simulink model "GTA_PCMFirmware"  (Simulink 7.8)
settings: Solver=FixedStepDiscrete  StartTime=0.0  StopTime=10.0  RelTol=1e-3
PreLoadFcn:
  | try, eval([bdroot '_setup']); catch, eval('model_setup', ''); end
InitFcn:
  | try, eval([bdroot '_setup']); catch, eval('model_setup', ''); end
undefined symbols (not defined in the file): fndFwd, fndNeut, fndRev, FWDlockout, GCM, keySwIgn2, motohawk_build_version, motohawk_trunc_name, motohawk_vardec_path, REVlockout
libraries: MotoHawk_lib x313, simulink x47, GTA_Library x13
(part 5 of 7)

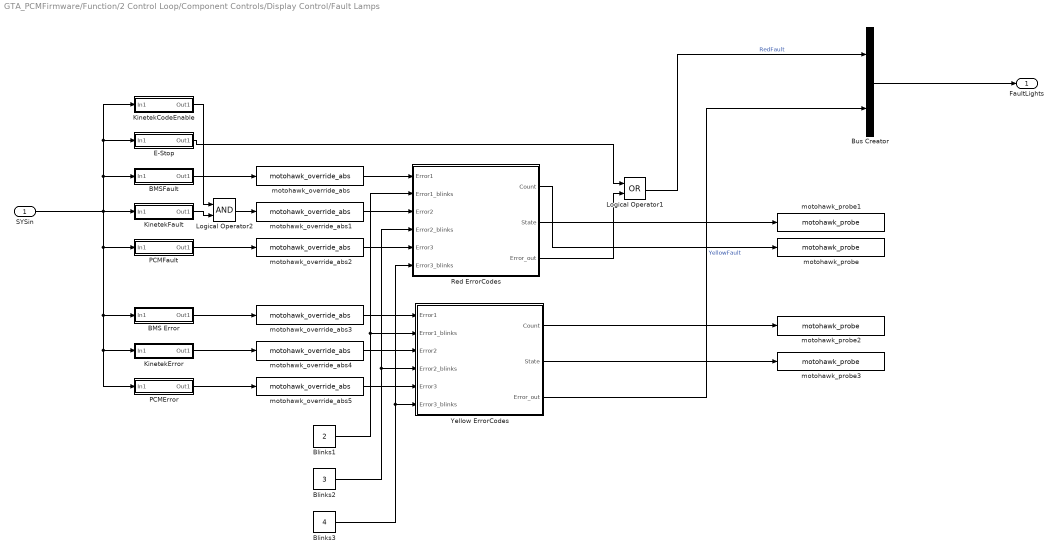
== system GTA_PCMFirmware/Function/2 Control Loop/Component Controls/Display Control/Fault Lamps ==
  SYSin : Inport
  BMS Error : Subsystem
  BMSFault : Subsystem
  Blinks1 : Constant  Value=2
  Blinks2 : Constant  Value=3
  Blinks3 : Constant  Value=4
  Bus Creator : BusCreator  Inputs=2
  E-Stop : Subsystem
  KinetekCodeEnable : Subsystem
  KinetekError : Subsystem
  KinetekFault : Subsystem
  Logical Operator1 : Logic  Operator=OR  AllPortsSameDT=off  OutDataTypeStr=boolean
  Logical Operator2 : Logic  AllPortsSameDT=off  OutDataTypeStr=boolean
  PCMError : Subsystem
  PCMFault : Subsystem
  Red ErrorCodes : Stateflow chart  TreatAsAtomicUnit=on
  Yellow ErrorCodes : Stateflow chart  TreatAsAtomicUnit=on
  motohawk_override_abs : MotoHawk_lib/Calibration & Probing Blocks/motohawk_override_abs  parent_name='BMSfltDBG'  parent_val=0  show_more=off  name_source=Use Parameter  parent_read_level=1  parent_override_level=1  view_as=Number  enum_struct={'Disabled', 'Enabled'}  use_help_units=off  parent_help=''  parent_units=''  use_min_max=off  parent_min=-inf  parent_max=inf  use_precision=off  parent_precision=''  parent_gain=1  parent_offset=0  parent_exp=1  use_mototune_group=off  parent_group=motohawk_vardec_path(gcb)
  motohawk_override_abs1 : MotoHawk_lib/Calibration & Probing Blocks/motohawk_override_abs  parent_name='KINETEKfltDBG'  parent_val=0  show_more=off  name_source=Use Parameter  parent_read_level=1  parent_override_level=1  view_as=Number  enum_struct={'Disabled', 'Enabled'}  use_help_units=off  parent_help=''  parent_units=''  use_min_max=off  parent_min=-inf  parent_max=inf  use_precision=off  parent_precision=''  parent_gain=1  parent_offset=0  parent_exp=1  use_mototune_group=off  parent_group=motohawk_vardec_path(gcb)
  motohawk_override_abs2 : MotoHawk_lib/Calibration & Probing Blocks/motohawk_override_abs  parent_name='PCMfltDBG'  parent_val=0  show_more=off  name_source=Use Parameter  parent_read_level=1  parent_override_level=1  view_as=Number  enum_struct={'Disabled', 'Enabled'}  use_help_units=off  parent_help=''  parent_units=''  use_min_max=off  parent_min=-inf  parent_max=inf  use_precision=off  parent_precision=''  parent_gain=1  parent_offset=0  parent_exp=1  use_mototune_group=off  parent_group=motohawk_vardec_path(gcb)
  motohawk_override_abs3 : MotoHawk_lib/Calibration & Probing Blocks/motohawk_override_abs  parent_name='BMSerrDBG'  parent_val=0  show_more=off  name_source=Use Parameter  parent_read_level=1  parent_override_level=1  view_as=Number  enum_struct={'Disabled', 'Enabled'}  use_help_units=off  parent_help=''  parent_units=''  use_min_max=off  parent_min=-inf  parent_max=inf  use_precision=off  parent_precision=''  parent_gain=1  parent_offset=0  parent_exp=1  use_mototune_group=off  parent_group=motohawk_vardec_path(gcb)
  motohawk_override_abs4 : MotoHawk_lib/Calibration & Probing Blocks/motohawk_override_abs  parent_name='KINETEKerrDBG'  parent_val=0  show_more=off  name_source=Use Parameter  parent_read_level=1  parent_override_level=1  view_as=Number  enum_struct={'Disabled', 'Enabled'}  use_help_units=off  parent_help=''  parent_units=''  use_min_max=off  parent_min=-inf  parent_max=inf  use_precision=off  parent_precision=''  parent_gain=1  parent_offset=0  parent_exp=1  use_mototune_group=off  parent_group=motohawk_vardec_path(gcb)
  motohawk_override_abs5 : MotoHawk_lib/Calibration & Probing Blocks/motohawk_override_abs  parent_name='PCMerrDBG'  parent_val=0  show_more=off  name_source=Use Parameter  parent_read_level=1  parent_override_level=1  view_as=Number  enum_struct={'Disabled', 'Enabled'}  use_help_units=off  parent_help=''  parent_units=''  use_min_max=off  parent_min=-inf  parent_max=inf  use_precision=off  parent_precision=''  parent_gain=1  parent_offset=0  parent_exp=1  use_mototune_group=off  parent_group=motohawk_vardec_path(gcb)
  motohawk_probe : MotoHawk_lib/Calibration & Probing Blocks/motohawk_probe  nam='Red_count'  show_more=off  name_source=Use Parameter  read_level=1  view_as=Number  enum_struct={'Disabled', 'Enabled'}  vector_style=Wide Row  use_help_units=off  help=''  units=''  use_header_enum=off  row_header_enum={}  col_header_enum={}  use_min_max=off  min_val=-inf  max_val=inf  use_precision=off  precision=''  gain=1  offset=0  exp=1  use_mototune_group=off  mototune_group=motohawk_vardec_path(gcb)
  motohawk_probe1 : MotoHawk_lib/Calibration & Probing Blocks/motohawk_probe  nam='Red_state'  show_more=off  name_source=Use Parameter  read_level=1  view_as=Number  enum_struct={'Disabled', 'Enabled'}  vector_style=Wide Row  use_help_units=off  help=''  units=''  use_header_enum=off  row_header_enum={}  col_header_enum={}  use_min_max=off  min_val=-inf  max_val=inf  use_precision=off  precision=''  gain=1  offset=0  exp=1  use_mototune_group=off  mototune_group=motohawk_vardec_path(gcb)
  motohawk_probe2 : MotoHawk_lib/Calibration & Probing Blocks/motohawk_probe  nam='Yellow_count'  show_more=off  name_source=Use Parameter  read_level=1  view_as=Number  enum_struct={'Disabled', 'Enabled'}  vector_style=Wide Row  use_help_units=off  help=''  units=''  use_header_enum=off  row_header_enum={}  col_header_enum={}  use_min_max=off  min_val=-inf  max_val=inf  use_precision=off  precision=''  gain=1  offset=0  exp=1  use_mototune_group=off  mototune_group=motohawk_vardec_path(gcb)
  motohawk_probe3 : MotoHawk_lib/Calibration & Probing Blocks/motohawk_probe  nam='Yellow_state'  show_more=off  name_source=Use Parameter  read_level=1  view_as=Number  enum_struct={'Disabled', 'Enabled'}  vector_style=Wide Row  use_help_units=off  help=''  units=''  use_header_enum=off  row_header_enum={}  col_header_enum={}  use_min_max=off  min_val=-inf  max_val=inf  use_precision=off  precision=''  gain=1  offset=0  exp=1  use_mototune_group=off  mototune_group=motohawk_vardec_path(gcb)
  FaultLights : Outport
  wires:
  SYSin/1 -> KinetekFault/1(In1), BMSFault/1(In1), E-Stop/1(In1), KinetekCodeEnable/1(In1), PCMFault/1(In1), BMS Error/1(In1), KinetekError/1(In1), PCMError/1(In1)
  Blinks1/1 -> Red ErrorCodes/2(Error1_blinks), Yellow ErrorCodes/2(Error1_blinks)
  Blinks2/1 -> Red ErrorCodes/4(Error2_blinks), Yellow ErrorCodes/4(Error2_blinks)
  Blinks3/1 -> Red ErrorCodes/6(Error3_blinks), Yellow ErrorCodes/6(Error3_blinks)
  BMSFault/1(Out1) -> motohawk_override_abs/1
  PCMFault/1(Out1) -> motohawk_override_abs2/1
  BMS Error/1(Out1) -> motohawk_override_abs3/1
  KinetekError/1(Out1) -> motohawk_override_abs4/1
  PCMError/1(Out1) -> motohawk_override_abs5/1
  E-Stop/1(Out1) -> Logical Operator1/1
  Yellow ErrorCodes/3(Error_out) -> Bus Creator/2  "YellowFault"
  Logical Operator1/1 -> Bus Creator/1  "RedFault"
  Red ErrorCodes/3(Error_out) -> Logical Operator1/2
  KinetekFault/1(Out1) -> Logical Operator2/2
  KinetekCodeEnable/1(Out1) -> Logical Operator2/1
  Logical Operator2/1 -> motohawk_override_abs1/1
  Yellow ErrorCodes/2(State) -> motohawk_probe3/1
  Yellow ErrorCodes/1(Count) -> motohawk_probe2/1
  Red ErrorCodes/2(State) -> motohawk_probe1/1
  Red ErrorCodes/1(Count) -> motohawk_probe/1
  motohawk_override_abs/1 -> Red ErrorCodes/1(Error1)
  motohawk_override_abs1/1 -> Red ErrorCodes/3(Error2)
  motohawk_override_abs2/1 -> Red ErrorCodes/5(Error3)
  motohawk_override_abs3/1 -> Yellow ErrorCodes/1(Error1)
  motohawk_override_abs4/1 -> Yellow ErrorCodes/3(Error2)
  motohawk_override_abs5/1 -> Yellow ErrorCodes/5(Error3)
  Bus Creator/1 -> FaultLights/1

== system GTA_PCMFirmware/Function/2 Control Loop/Component Controls/Display Control/Gearbox Display ==
  SYSin : Inport
  MotorControl : Inport  Port=2
  Bus Selector : BusSelector  OutputSignals=fndOutput
  Bus Selector1 : BusSelector  OutputSignals=ModeControl.StatusBits.DriveMode
  Data Type Conversion : DataTypeConversion  OutDataTypeStr=boolean
  Drive : Constant  Value=hex2dec('B')  OutDataTypeStr=uint16
  DriveOrRev : Constant  OutDataTypeStr=boolean
  Flash Neutral : Constant  Value=hex2dec('C')  OutDataTypeStr=uint16
  Logical Operator : Logic  Operator=NOT  AllPortsSameDT=off  OutDataTypeStr=boolean
  Logical Operator1 : Logic  Inputs=3  AllPortsSameDT=off  OutDataTypeStr=boolean
  Multiport Switch : MultiPortSwitch  DataPortOrder=Zero-based contiguous  Inputs=4  zeroidx=on
  Multiport Switch1 : MultiPortSwitch  DataPortOrder=Zero-based contiguous  Inputs=4  zeroidx=on
  Multiport Switch2 : MultiPortSwitch  DataPortOrder=Zero-based contiguous  Inputs=2  zeroidx=on
  Neutral : Constant  Value=hex2dec('C')  OutDataTypeStr=uint16
  Neutral1 : Constant  Value=0  OutDataTypeStr=boolean
  NotValid : Constant  Value=hex2dec('F')  OutDataTypeStr=uint16
  Pulse Generator : DiscretePulseGenerator  Period=250  PulseWidth=125  SampleTime=-1
  Reverse : Constant  Value=hex2dec('D')  OutDataTypeStr=uint16
  GboxPos : Outport
  wires:
  MotorControl/1 -> Bus Selector/1
  Bus Selector/1 -> Multiport Switch/1, Multiport Switch1/1  "<fndOutput>"
  Neutral/1 -> Multiport Switch/2
  NotValid/1 -> Multiport Switch/5
  Multiport Switch/1 -> Multiport Switch2/2  "GearboxPositionIPC"
  Reverse/1 -> Multiport Switch/3
  Drive/1 -> Multiport Switch/4
  DriveOrRev/1 -> Multiport Switch1/3, Multiport Switch1/4
  Neutral1/1 -> Multiport Switch1/2, Multiport Switch1/5
  Bus Selector1/1 -> Logical Operator/1  "<DriveMode>"
  Multiport Switch1/1 -> Logical Operator1/1
  Logical Operator/1 -> Logical Operator1/2
  Pulse Generator/1 -> Data Type Conversion/1
  Logical Operator1/1 -> Multiport Switch2/1
  Flash Neutral/1 -> Multiport Switch2/3
  Multiport Switch2/1 -> GboxPos/1  "GearboxPositionIPC"
  Data Type Conversion/1 -> Logical Operator1/3
  SYSin/1 -> Bus Selector1/1

== system GTA_PCMFirmware/Function/2 Control Loop/Component Controls/Display Control/ReadyLight ==
  SYSin : Inport
  Bus Selector1 : BusSelector  OutputSignals=ReadyState,ModeControl.StatusBits.ReadyOk
  Logical Operator : Logic  AllPortsSameDT=off  OutDataTypeStr=boolean
  ReadyLight : Outport
  wires:
  SYSin/1 -> Bus Selector1/1
  Bus Selector1/1 -> Logical Operator/1  "<ReadyState>"
  Bus Selector1/2 -> Logical Operator/2  "<ReadyOk>"
  Logical Operator/1 -> ReadyLight/1

== system GTA_PCMFirmware/Function/2 Control Loop/Component Controls/Display Control/Vehicle Speed ==
  SYSin : Inport
  Bus Selector1 : BusSelector  OutputSignals=BUS.Input Bus.CANin.Motor Controller.KinVoltSpeed.SpeedLPF
  RPMtoInperMin : Gain  Gain=33/4925  OutDataTypeStr=single
  Out1 : Outport
  wires:
  SYSin/1 -> Bus Selector1/1
  Bus Selector1/1 -> RPMtoInperMin/1  "<SpeedLPF>"
  RPMtoInperMin/1 -> Out1/1  "vehSpeed"

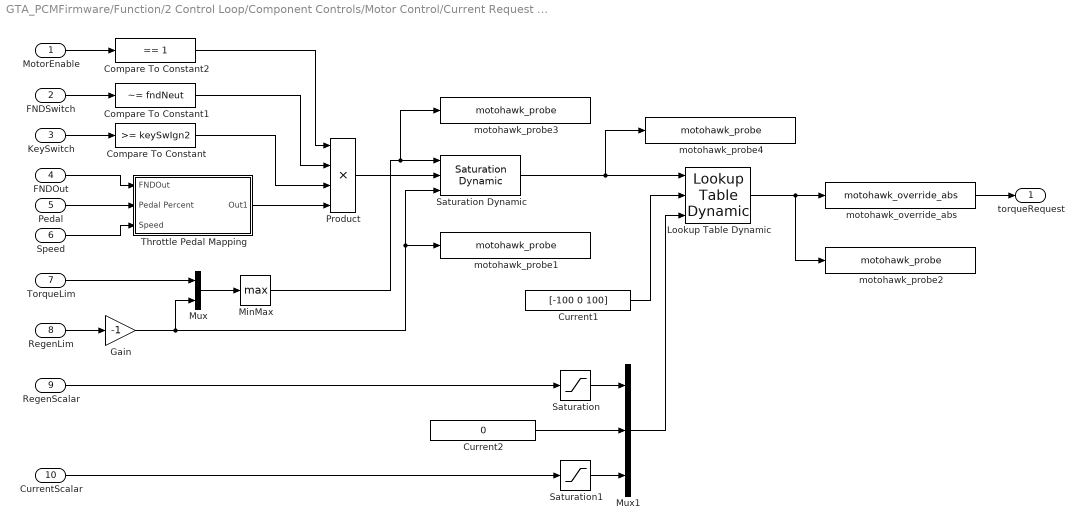
== system GTA_PCMFirmware/Function/2 Control Loop/Component Controls/Motor Control/Current Request Algorithm ==
  MotorEnable : Inport
  "FNDSwitch " : Inport  Port=2
  KeySwitch : Inport  Port=3
  FNDOut : Inport  Port=4
  "Pedal " : Inport  Port=5
  Speed : Inport  Port=6
  "TorqueLim " : Inport  Port=7
  RegenLim : Inport  Port=8
  RegenScalar : Inport  Port=9  OutDataTypeStr=single
  CurrentScalar : Inport  Port=10  OutDataTypeStr=single
  Compare To Constant : simulink/Logic and Bit Operations/Compare To Constant  relop=>=  const=keySwIgn2  OutDataTypeStr=uint8
  Compare To Constant1 : simulink/Logic and Bit Operations/Compare To Constant  relop=~=  const=fndNeut  OutDataTypeStr=uint8
  Compare To Constant2 : simulink/Logic and Bit Operations/Compare To Constant  relop===  const=1  OutDataTypeStr=uint8
  Current1 : Constant  Value=[-100 0 100]  OutDataTypeStr=single
  Current2 : Constant  Value=0  OutDataTypeStr=single
  Gain : Gain  Gain=-1
  Lookup Table Dynamic : simulink/Lookup Tables/Lookup Table Dynamic  LookUpMeth=Interpolation-Use End Values  OutDataTypeStr=fixdt('single')  OutputDataTypeScalingMode=Specify via dialog  OutDataType=fixdt('single')  OutScaling=[]  DoSatur=off
  MinMax : MinMax  Function=max
  Mux : Mux  Inputs=2
  Mux1 : Mux  Inputs=3
  Product : Product  Inputs=4  OutDataTypeStr=single  RndMeth=Zero
  Saturation : Saturate  UpperLimit=0  LowerLimit=-1000  OutDataTypeStr=single
  Saturation Dynamic : simulink/Discontinuities/Saturation Dynamic  OutMin=[]  OutMax=[]  OutDataTypeStr=Inherit: Same as second input  OutDataType=fixdt(1, 16)  OutScaling=2^-10  DoSatur=off
  Saturation1 : Saturate  UpperLimit=1000  LowerLimit=0  OutDataTypeStr=single
  Throttle Pedal Mapping : Subsystem
  motohawk_override_abs : MotoHawk_lib/Calibration & Probing Blocks/motohawk_override_abs  parent_name='Motor_Current_Override'  parent_val=0  show_more=on  name_source=Use Parameter  parent_read_level=1  parent_override_level=1  view_as=Number  enum_struct={'Disabled', 'Enabled'}  use_help_units=off  parent_help=''  parent_units=''  use_min_max=off  parent_min=-inf  parent_max=inf  use_precision=off  parent_precision=''  parent_gain=1  parent_offset=0  parent_exp=1  use_mototune_group=off  parent_group=motohawk_vardec_path(gcb)
  motohawk_probe1 : MotoHawk_lib/Calibration & Probing Blocks/motohawk_probe  nam='LowSatLimit'  show_more=on  name_source=Use Parameter  read_level=1  view_as=Number  enum_struct={'Disabled', 'Enabled'}  vector_style=Wide Row  use_help_units=off  help=''  units=''  use_header_enum=off  row_header_enum={}  col_header_enum={}  use_min_max=off  min_val=-inf  max_val=inf  use_precision=off  precision=''  gain=1  offset=0  exp=1  use_mototune_group=off  mototune_group=motohawk_vardec_path(gcb)
  motohawk_probe2 : MotoHawk_lib/Calibration & Probing Blocks/motohawk_probe  nam='Motor_Current_Output'  show_more=on  name_source=Use Parameter  read_level=1  view_as=Number  enum_struct={'Disabled', 'Enabled'}  vector_style=Wide Row  use_help_units=off  help=''  units=''  use_header_enum=off  row_header_enum={}  col_header_enum={}  use_min_max=off  min_val=-inf  max_val=inf  use_precision=off  precision=''  gain=1  offset=0  exp=1  use_mototune_group=off  mototune_group=motohawk_vardec_path(gcb)
  motohawk_probe3 : MotoHawk_lib/Calibration & Probing Blocks/motohawk_probe  nam='HighSatLimit'  show_more=on  name_source=Use Parameter  read_level=1  view_as=Number  enum_struct={'Disabled', 'Enabled'}  vector_style=Wide Row  use_help_units=off  help=''  units=''  use_header_enum=off  row_header_enum={}  col_header_enum={}  use_min_max=off  min_val=-inf  max_val=inf  use_precision=off  precision=''  gain=1  offset=0  exp=1  use_mototune_group=off  mototune_group=motohawk_vardec_path(gcb)
  motohawk_probe4 : MotoHawk_lib/Calibration & Probing Blocks/motohawk_probe  nam='PedalLookupOutPercent'  show_more=on  name_source=Use Parameter  read_level=1  view_as=Number  enum_struct={'Disabled', 'Enabled'}  vector_style=Wide Row  use_help_units=off  help=''  units=''  use_header_enum=off  row_header_enum={}  col_header_enum={}  use_min_max=off  min_val=-inf  max_val=inf  use_precision=off  precision=''  gain=1  offset=0  exp=1  use_mototune_group=off  mototune_group=motohawk_vardec_path(gcb)
  torqueRequest : Outport
  wires:
  "TorqueLim "/1 -> Mux/1
  KeySwitch/1 -> Compare To Constant/1
  "FNDSwitch "/1 -> Compare To Constant1/1
  motohawk_override_abs/1 -> torqueRequest/1
  FNDOut/1 -> Throttle Pedal Mapping/1(FNDOut)
  "Pedal "/1 -> Throttle Pedal Mapping/2(Pedal Percent)
  Speed/1 -> Throttle Pedal Mapping/3(Speed)
  Throttle Pedal Mapping/1(Out1) -> Product/4
  Compare To Constant/1 -> Product/3
  Compare To Constant1/1 -> Product/2
  Product/1 -> Saturation Dynamic/2
  Mux/1 -> MinMax/1
  MinMax/1 -> motohawk_probe3/1, Saturation Dynamic/1
  Lookup Table Dynamic/1 -> motohawk_override_abs/1, motohawk_probe2/1
  Saturation Dynamic/1 -> Lookup Table Dynamic/1, motohawk_probe4/1
  RegenLim/1 -> Gain/1
  Current1/1 -> Lookup Table Dynamic/2
  Saturation/1 -> Mux1/1
  Current2/1 -> Mux1/2
  Saturation1/1 -> Mux1/3
  Mux1/1 -> Lookup Table Dynamic/3
  RegenScalar/1 -> Saturation/1
  Gain/1 -> Mux/2, Saturation Dynamic/3, motohawk_probe1/1
  MotorEnable/1 -> Compare To Constant2/1
  Compare To Constant2/1 -> Product/1
  CurrentScalar/1 -> Saturation1/1

== system GTA_PCMFirmware/Function/2 Control Loop/Component Controls/Motor Control/Direction Lockout ==
  " FNDSw" : Inport
  " Speed" : Inport  Port=2
  Forward : simulink/Logic and Bit Operations/Compare To Constant  relop===  const=fndRev  OutDataTypeStr=boolean
  Fwd Lockout : simulink/Logic and Bit Operations/Compare To Constant  relop=>=  const=FWDlockout  OutDataTypeStr=boolean
  Fwd while Rev : Logic  AllPortsSameDT=off  OutDataTypeStr=boolean
  Gain : Gain  OutDataTypeStr=uint16
  Multiport Switch : MultiPortSwitch  DataPortOrder=Specify indices  Inputs=2  DataPortIndices={0,1}  zeroidx=off
  Neutral : Constant  Value=fndNeut
  Neutral command : Logic  Operator=OR  AllPortsSameDT=off  OutDataTypeStr=boolean
  Rev Lockout : simulink/Logic and Bit Operations/Compare To Constant  relop=<=  const=REVlockout  OutDataTypeStr=boolean
  Rev while Fwd : Logic  AllPortsSameDT=off  OutDataTypeStr=boolean
  Reverse : simulink/Logic and Bit Operations/Compare To Constant  relop===  const=fndFwd  OutDataTypeStr=boolean
  " FNDOut" : Outport
  wires:
  " FNDSw"/1 -> Gain/1
  Gain/1 -> Forward/1, Reverse/1, Multiport Switch/2  "fndOutput"
  " Speed"/1 -> Fwd Lockout/1, Rev Lockout/1
  Forward/1 -> Rev while Fwd/1
  Fwd Lockout/1 -> Rev while Fwd/2
  Reverse/1 -> Fwd while Rev/1
  Rev Lockout/1 -> Fwd while Rev/2
  Fwd while Rev/1 -> Neutral command/2
  Rev while Fwd/1 -> Neutral command/1
  Multiport Switch/1 -> " FNDOut"/1  "fndOutput"
  Neutral/1 -> Multiport Switch/3
  Neutral command/1 -> Multiport Switch/1

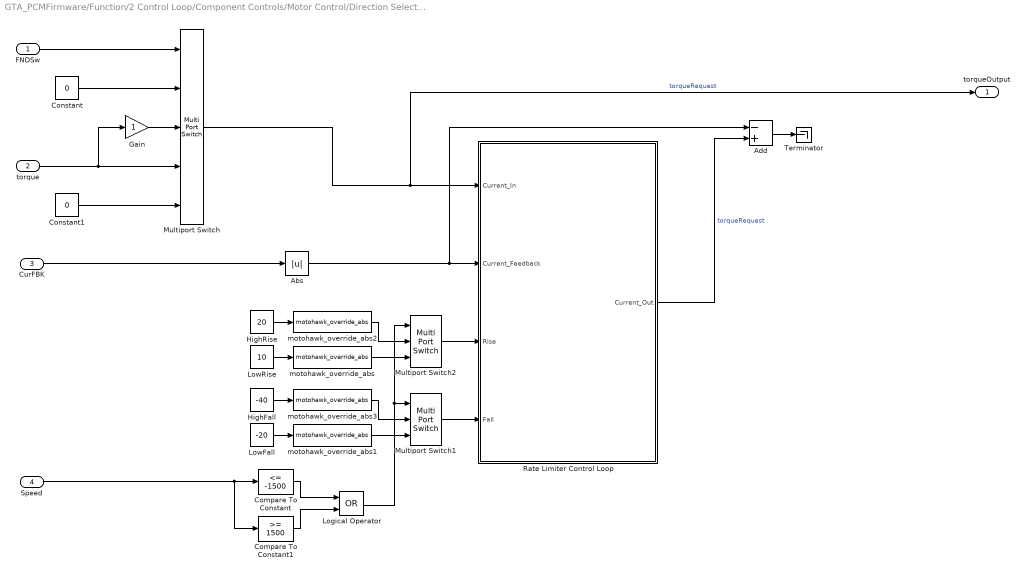
== system GTA_PCMFirmware/Function/2 Control Loop/Component Controls/Motor Control/Direction Selector & Control Loop ==
  " FNDSw" : Inport
  " torque" : Inport  Port=2
  CurFBK : Inport  Port=3
  Speed : Inport  Port=4
  Abs : Abs
  Add : Sum  Inputs=-+
  Compare To Constant : simulink/Logic and Bit Operations/Compare To Constant  relop=<=  const=-1500  OutDataTypeStr=boolean
  Compare To Constant1 : simulink/Logic and Bit Operations/Compare To Constant  relop=>=  const=1500  OutDataTypeStr=boolean
  Constant : Constant  Value=0
  Constant1 : Constant  Value=0
  Gain : Gain
  HighFall : Constant  Value=-40
  HighRise : Constant  Value=20
  Logical Operator : Logic  Operator=OR  AllPortsSameDT=off  OutDataTypeStr=boolean
  LowFall : Constant  Value=-20
  LowRise : Constant  Value=10
  Multiport Switch : MultiPortSwitch  DataPortOrder=Zero-based contiguous  Inputs=4  zeroidx=on
  Multiport Switch1 : MultiPortSwitch  DataPortOrder=Specify indices  DataPortIndices={1,0}  zeroidx=off
  Multiport Switch2 : MultiPortSwitch  DataPortOrder=Specify indices  DataPortIndices={1,0}  zeroidx=off
  Rate Limiter Control Loop : Stateflow chart  TreatAsAtomicUnit=on
  Terminator : Terminator
  motohawk_override_abs : MotoHawk_lib/Calibration & Probing Blocks/motohawk_override_abs  parent_name='RateLimitRiseLow'  parent_val=10  show_more=off  name_source=Use Parameter  parent_read_level=1  parent_override_level=1  view_as=Number  enum_struct={'Disabled', 'Enabled'}  use_help_units=off  parent_help=''  parent_units=''  use_min_max=off  parent_min=-inf  parent_max=inf  use_precision=off  parent_precision=''  parent_gain=1  parent_offset=0  parent_exp=1  use_mototune_group=off  parent_group=motohawk_vardec_path(gcb)
  motohawk_override_abs1 : MotoHawk_lib/Calibration & Probing Blocks/motohawk_override_abs  parent_name='RateLimitFallLow'  parent_val=0  show_more=off  name_source=Use Parameter  parent_read_level=1  parent_override_level=1  view_as=Number  enum_struct={'Disabled', 'Enabled'}  use_help_units=off  parent_help=''  parent_units=''  use_min_max=off  parent_min=-inf  parent_max=inf  use_precision=off  parent_precision=''  parent_gain=1  parent_offset=0  parent_exp=1  use_mototune_group=off  parent_group=motohawk_vardec_path(gcb)
  motohawk_override_abs2 : MotoHawk_lib/Calibration & Probing Blocks/motohawk_override_abs  parent_name='RateLimitRiseHigh'  parent_val=10  show_more=off  name_source=Use Parameter  parent_read_level=1  parent_override_level=1  view_as=Number  enum_struct={'Disabled', 'Enabled'}  use_help_units=off  parent_help=''  parent_units=''  use_min_max=off  parent_min=-inf  parent_max=inf  use_precision=off  parent_precision=''  parent_gain=1  parent_offset=0  parent_exp=1  use_mototune_group=off  parent_group=motohawk_vardec_path(gcb)
  motohawk_override_abs3 : MotoHawk_lib/Calibration & Probing Blocks/motohawk_override_abs  parent_name='RateLimitFallHigh'  parent_val=0  show_more=off  name_source=Use Parameter  parent_read_level=1  parent_override_level=1  view_as=Number  enum_struct={'Disabled', 'Enabled'}  use_help_units=off  parent_help=''  parent_units=''  use_min_max=off  parent_min=-inf  parent_max=inf  use_precision=off  parent_precision=''  parent_gain=1  parent_offset=0  parent_exp=1  use_mototune_group=off  parent_group=motohawk_vardec_path(gcb)
  torqueOutput : Outport
  wires:
  " FNDSw"/1 -> Multiport Switch/1
  " torque"/1 -> Multiport Switch/4, Gain/1
  Gain/1 -> Multiport Switch/3
  Constant/1 -> Multiport Switch/2
  Constant1/1 -> Multiport Switch/5
  Speed/1 -> Compare To Constant/1, Compare To Constant1/1
  Compare To Constant/1 -> Logical Operator/1
  Compare To Constant1/1 -> Logical Operator/2
  Multiport Switch/1 -> Rate Limiter Control Loop/1(Current_In), torqueOutput/1  "torqueRequest"
  LowFall/1 -> motohawk_override_abs1/1
  LowRise/1 -> motohawk_override_abs/1
  HighRise/1 -> motohawk_override_abs2/1
  HighFall/1 -> motohawk_override_abs3/1
  motohawk_override_abs/1 -> Multiport Switch2/3
  motohawk_override_abs1/1 -> Multiport Switch1/3
  motohawk_override_abs3/1 -> Multiport Switch1/2
  motohawk_override_abs2/1 -> Multiport Switch2/2
  Multiport Switch2/1 -> Rate Limiter Control Loop/3(Rise)
  Multiport Switch1/1 -> Rate Limiter Control Loop/4(Fall)
  Logical Operator/1 -> Multiport Switch2/1, Multiport Switch1/1
  CurFBK/1 -> Abs/1
  Rate Limiter Control Loop/1(Current_Out) -> Add/2  "torqueRequest"
  Abs/1 -> Rate Limiter Control Loop/2(Current_Feedback), Add/1
  Add/1 -> Terminator/1

== system GTA_PCMFirmware/Function/2 Control Loop/Component Controls/Motor Control/Enable ==
  "driveEnable " : Inport
  errorField : Inport  Port=2
  Compare To Constant : simulink/Logic and Bit Operations/Compare To Constant  relop===  const=0  OutDataTypeStr=uint8
  Logical Operator : Logic  AllPortsSameDT=off  OutDataTypeStr=boolean
  Terminator : Terminator
  enable : Outport
  wires:
  Logical Operator/1 -> enable/1  "enable"
  "driveEnable "/1 -> Logical Operator/1, Logical Operator/2
  errorField/1 -> Compare To Constant/1
  Compare To Constant/1 -> Terminator/1

== system GTA_PCMFirmware/Function/2 Control Loop/Mode Control & Ready/Mode Control/Status Bits ==
  ModeState : Inport
  Fault_ID : Inport  Port=2
  HVstate : Inport  Port=3
  ACC2Mode : simulink/Logic and Bit Operations/Compare To Constant  relop=~=  const=0  OutDataTypeStr=uint8
  Bus Creator : BusCreator  Inputs=6
  Compare : simulink/Logic and Bit Operations/Compare To Constant  relop===  const=2  OutDataTypeStr=uint8
  Compare1 : simulink/Logic and Bit Operations/Compare To Constant  relop===  const=1  OutDataTypeStr=uint8
  Compare2 : simulink/Logic and Bit Operations/Compare To Constant  relop===  const=5  OutDataTypeStr=uint8
  Compare3 : simulink/Logic and Bit Operations/Compare To Constant  relop=~=  const=0  OutDataTypeStr=uint8
  Compare4 : simulink/Logic and Bit Operations/Compare To Constant  relop===  const=4  OutDataTypeStr=uint8
  Compare5 : simulink/Logic and Bit Operations/Compare To Constant  relop===  const=2  OutDataTypeStr=uint8
  Logical Operator : Logic  Operator=OR  AllPortsSameDT=off  OutDataTypeStr=boolean
  Terminator : Terminator
  StatusOut : Outport
  wires:
  Bus Creator/1 -> StatusOut/1
  Compare1/1 -> Logical Operator/1
  Compare/1 -> Logical Operator/2
  Logical Operator/1 -> Bus Creator/1  "ChargeMode"
  Compare2/1 -> Bus Creator/2  "DriveMode"
  Fault_ID/1 -> Compare3/1, Compare4/1, Compare5/1
  Compare3/1 -> Bus Creator/3  "FaultMode"
  ModeState/1 -> Compare1/1, Compare/1, Compare2/1, ACC2Mode/1
  Compare4/1 -> Bus Creator/4  "ContactorFault"
  Compare5/1 -> Bus Creator/5  "BatteryFault"
  ACC2Mode/1 -> Bus Creator/6  "ReadyOk"
  HVstate/1 -> Terminator/1

== system GTA_PCMFirmware/Function/2 Control Loop/Safety/Current Limit/RegenLimit ==
  InputBus : Inport
  Bus Creator : BusCreator  Inputs=3
  Cell Temp too high : simulink/Logic and Bit Operations/Compare To Zero  relop===  OutDataTypeStr=uint8
  Cell Temp too low : simulink/Logic and Bit Operations/Compare To Zero  relop===  OutDataTypeStr=uint8
  Cell Voltage limiter : Subsystem
  Current Limiter : Subsystem
  High Cell Temp : Subsystem
  Low Cell Temp : Subsystem
  MinMax : MinMax
  Mux : Mux  Inputs=6
  Pack Voltage Limiter : Subsystem
  SOC Limiter : Subsystem
  Saturation : Saturate  UpperLimit=100  LowerLimit=0  OutDataTypeStr=single
  motohawk_probe : MotoHawk_lib/Calibration & Probing Blocks/motohawk_probe  nam='RegenLimitPerc'  show_more=off  name_source=Use Parameter  read_level=1  view_as=Number  enum_struct={'Disabled', 'Enabled'}  vector_style=Wide Row  use_help_units=off  help=''  units=''  use_header_enum=off  row_header_enum={}  col_header_enum={}  use_min_max=off  min_val=-inf  max_val=inf  use_precision=off  precision=''  gain=1  offset=0  exp=1  use_mototune_group=off  mototune_group=motohawk_vardec_path(gcb)
  Out : Outport
  wires:
  InputBus/1 -> SOC Limiter/1(InputBus), Pack Voltage Limiter/1(InputBus), Current Limiter/1(InputBus), Cell Voltage limiter/1(InputBus), Low Cell Temp/1(InputBus), High Cell Temp/1(InputBus)
  Pack Voltage Limiter/1(PercOut) -> Mux/1
  Current Limiter/1(PercOut) -> Mux/2
  SOC Limiter/1(PercOut) -> Mux/3
  Mux/1 -> Saturation/1
  Bus Creator/1 -> Out/1
  Saturation/1 -> MinMax/1, motohawk_probe/1
  MinMax/1 -> Bus Creator/1  "MaxRegenPerc"
  Cell Temp too low/1 -> Bus Creator/3  "CellRegTempLo"
  Cell Temp too high/1 -> Bus Creator/2  "CellRegTempHi"
  Cell Voltage limiter/1(PercOut) -> Mux/4
  High Cell Temp/1(PercOut) -> Mux/5, Cell Temp too high/1
  Low Cell Temp/1(PercOut) -> Mux/6, Cell Temp too low/1

== system GTA_PCMFirmware/Function/2 Control Loop/Safety/Current Limit/TorqueLimit ==
  InputBus : Inport
  Bus Creator : BusCreator  Inputs=3
  Cell Temp too high : simulink/Logic and Bit Operations/Compare To Zero  relop===  OutDataTypeStr=uint8
  Cell Temp too low : simulink/Logic and Bit Operations/Compare To Zero  relop===  OutDataTypeStr=uint8
  Cell Voltage limiter : Subsystem
  Current Limiter : Subsystem
  High Cell Temp : Subsystem
  Low Cell Temp : Subsystem
  MinMax : MinMax
  Mux : Mux  Inputs=7
  Pack Voltage Limiter : Subsystem
  SOC Limiter : Subsystem
  Saturation : Saturate  UpperLimit=100  LowerLimit=-100  OutDataTypeStr=single
  Speed Limiter : Subsystem
  motohawk_probe : MotoHawk_lib/Calibration & Probing Blocks/motohawk_probe  nam='torqueLimitPerc'  show_more=off  name_source=Use Parameter  read_level=1  view_as=Number  enum_struct={'Disabled', 'Enabled'}  vector_style=Wide Row  use_help_units=off  help=''  units=''  use_header_enum=off  row_header_enum={}  col_header_enum={}  use_min_max=off  min_val=-inf  max_val=inf  use_precision=off  precision=''  gain=1  offset=0  exp=1  use_mototune_group=off  mototune_group=motohawk_vardec_path(gcb)
  Out : Outport
  wires:
  InputBus/1 -> Speed Limiter/1(InputBus), SOC Limiter/1(InputBus), Pack Voltage Limiter/1(InputBus), Current Limiter/1(InputBus), Low Cell Temp/1(InputBus), High Cell Temp/1(InputBus), Cell Voltage limiter/1(InputBus)
  Pack Voltage Limiter/1(PercOut) -> Mux/1
  Current Limiter/1(PercOut) -> Mux/2
  SOC Limiter/1(PercOut) -> Mux/3
  Speed Limiter/1(PercentOut) -> Mux/4
  Cell Voltage limiter/1(PercOut) -> Mux/5
  High Cell Temp/1(PercOut) -> Mux/6, Cell Temp too high/1
  Low Cell Temp/1(PercOut) -> Mux/7, Cell Temp too low/1
  Mux/1 -> Saturation/1
  Bus Creator/1 -> Out/1
  Saturation/1 -> MinMax/1, motohawk_probe/1
  MinMax/1 -> Bus Creator/1  "MaxCurrPerc"
  Cell Temp too low/1 -> Bus Creator/3  "CellDisTempLo"
  Cell Temp too high/1 -> Bus Creator/2  "CellDisTempHi"

== system GTA_PCMFirmware/Function/2 Control Loop/Safety/Faults/BatteryFault ==
  InputBus : Inport
  {1,4..5,7} (4 alike) : RelationalOperator  OutDataTypeStr=boolean
  {2..3,6,8} (4 alike) : RelationalOperator  Operator=<=  OutDataTypeStr=boolean
  Bus Creator : BusCreator  Inputs=2
  Bus Creator1 : BusCreator  Inputs=8
  Bus Selector : BusSelector  OutputSignals=Input Bus.CANin.BMS.csCellInfo.PackVoltage,Input Bus.Limits.BattLimits.MaxPackVoltage,Input Bus.CANin.BMS.csCellInfo.PackVoltage,Input Bus.Limits.BattLimits.MinPackVoltage,Input Bus.CANin.BMS.csInfo.csCurrent,Input Bus.Limits.BattLimits.CurrentLimit,Input Bus.CANin.BMS.csInfo.csCurrent,Input Bus.Limits.BattLimits.RegenLimit,Input Bus.CANin.BMS.csCellInfo.HighCellValue,Input Bus.Limits.BattLimits.MaxCellVoltage,Input Bus.CANin.BMS.csCellInfo.LowCellValue,Input Bus.Limits.BattLimits.MinCellVoltage,Input Bus.CANin.BMS.csCellTemps.HighCellTemp,Input Bus.Limits.BattLimits.BFmaxCellTemp,Input Bus.CANin.BMS.csCellTemps.LowCellTemp,Input Bus.Limits.BattLimits.BFminCellTemp
  Filter : Subsystem
  Logical Operator : Logic  Operator=OR  Inputs=1  AllPortsSameDT=off  OutDataTypeStr=boolean
  Mux : Mux  Inputs=8
  motohawk_probe : MotoHawk_lib/Calibration & Probing Blocks/motohawk_probe  nam='battFault'  show_more=off  name_source=Use Parameter  read_level=1  view_as=Number  enum_struct={'Disabled', 'Enabled'}  vector_style=Wide Row  use_help_units=off  help=''  units=''  use_header_enum=off  row_header_enum={}  col_header_enum={}  use_min_max=off  min_val=-inf  max_val=inf  use_precision=off  precision=''  gain=1  offset=0  exp=1  use_mototune_group=off  mototune_group=motohawk_vardec_path(gcb)
  BatteryFault : Outport
  wires:
  InputBus/1 -> Bus Selector/1
  Bus Selector/6 -> 3/2  "<CurrentLimit>"
  Bus Selector/8 -> 4/2  "<RegenLimit>"
  Bus Selector/9 -> 5/1  "<HighCellValue>"
  Bus Selector/10 -> 5/2  "<MaxCellVoltage>"
  Bus Selector/11 -> 6/1  "<LowCellValue>"
  Bus Selector/12 -> 6/2  "<MinCellVoltage>"
  Bus Selector/2 -> 1/2  "<MaxPackVoltage>"
  Bus Selector/4 -> 2/2  "<MinPackVoltage>"
  1/1 -> Mux/1, Bus Creator1/1  "PackVoltHigh"
  6/1 -> Mux/6, Bus Creator1/6  "CellVoltLow"
  5/1 -> Mux/5, Bus Creator1/5  "CellVoltHigh"
  4/1 -> Mux/4, Bus Creator1/4  "PackOverRegen"
  3/1 -> Mux/3, Bus Creator1/3  "PackOverCurrent"
  2/1 -> Mux/2, Bus Creator1/2  "PackVoltLow"
  Mux/1 -> Logical Operator/1, motohawk_probe/1
  Logical Operator/1 -> Filter/1(In1)
  Bus Creator1/1 -> Bus Creator/2  "BatteryFaultDBG"
  Bus Creator/1 -> BatteryFault/1
  Bus Selector/1 -> 1/1  "<PackVoltage>"
  Bus Selector/3 -> 2/1  "<PackVoltage>"
  Bus Selector/7 -> 4/1  "<csCurrent>"
  Bus Selector/5 -> 3/1  "<csCurrent>"
  Bus Selector/13 -> 7/1  "<HighCellTemp>"
  Bus Selector/14 -> 7/2  "<BFmaxCellTemp>"
  Bus Selector/15 -> 8/1  "<LowCellTemp>"
  Bus Selector/16 -> 8/2  "<BFminCellTemp>"
  8/1 -> Mux/8, Bus Creator1/8  "CellTempLow"
  7/1 -> Mux/7, Bus Creator1/7  "CellTempHigh"
  Filter/1(Out1) -> Bus Creator/1  "BatteryFault"

== system GTA_PCMFirmware/Function/3 Output and Debug/CAN/Debug/Message 0x700 ==
  In1 : Inport
  Bus Selector : BusSelector  OutputSignals=InputBus.DigitalIn.EStop,DebugBus.IGN1,InputBus.DigitalIn.KeySwitch.dbgKeySW.dbgIGN2,InputBus.DigitalIn.KeySwitch.dbgKeySW.dbgCrank,InputBus.DigitalIn.Shifter.dbgShifter.dbgShiftN,InputBus.DigitalIn.Shifter.dbgShifter.dbgShiftR,InputBus.DigitalIn.Shifter.dbgShifter.dbgShiftF,InputBus.DigitalIn.Shifter.dbgShifter.sbgShiftErr,InputBus.DigitalIn.BrakeSwitch.BrakeSw,InputBus.DigitalIn.RearDefrostSw.DefrostSW,InputBus.DigitalIn.WiperSw.WiperSw,InputBus.AnalogIn.ThrottlePedal.dbgAPPok,InputBus.CANin.BMS.csInfo.csCANok,InputBus.CANin.Motor Controller.KinCurrFB.CurrentFdbkOK,InputBus.CANin.Charger.CANchargerOK,DebugBus.SOCok,InputBus.CANin.Motor Controller.KinVoltSpeed.ErrorField,ControlBus.SYSin.BUS.Faults.BatteryFault.BatteryFault,ControlBus.SYSin.BUS.Faults.BatteryFault.BatteryFaultDBG.PackVoltLow,ControlBus.SYSin.BUS.Faults.BatteryFault.BatteryFaultDBG.PackOverCurrent,ControlBus.SYSin.BUS.Faults.BatteryFault.BatteryFaultDBG.PackOverRegen,ControlBus.SYSin.BUS.Faults.BatteryFault.BatteryFaultDBG.CellVoltHigh,ControlBus.SYSin.BUS.Faults.BatteryFault.BatteryFaultDBG.CellVoltLow,ControlBus.SYSin.BUS.Voltage level.VoltageFault,ControlBus.Display.ReadyLight,ControlBus.SYSin.ModeControl.StatusBits.FaultMode,ControlBus.SYSin.ModeControl.StatusBits.DriveMode,ControlBus.SYSin.ModeControl.StatusBits.ChargeMode,InputBus.DigitalIn.Charger.acPresent,DebugBus.DBGinverterOT,DebugBus.DBGmotorOT,ControlBus.SYSin.ModeControl.StatusBits.BatteryFault,InputBus.CANin.Charger.Charger Enabled,ControlBus.Charger.ChargerOut,InputBus.CANin.BMS.csChargeFlags.PackBalanced,InputBus.CANin.BMS.csChargeFlags.PackCharging,InputBus.CANin.BMS.csChargeFlags.PackCooldown,InputBus.CANin.BMS.csChargeFlags.PackCharged,InputBus.CANin.BMS.csChargeFlags.CellDrained,InputBus.CANin.BMS.csChargeFlags.CellsCharged,InputBus.CANin.BMS.csChargeFlags.CellOver,InputBus.CANin.BMS.csChargeFlags.CellHigh,ControlBus.SYSin.ModeControl.StatusBits.ContactorFault,ControlBus.SYSin.ModeControl.SSCont,ControlBus.SYSin.ModeControl.MainCont,ControlBus.SYSin.ModeControl.HVaccRly
  Send CAN Messages : MotoHawk_lib/CAN Blocks/Send CAN Messages  bus=-2  nam='CAN_1'  msgl=CANMSG_Debug700  pace=5  labelwires=off
  wires:
  In1/1 -> Bus Selector/1
  Bus Selector/1 -> Send CAN Messages/1  "<EStop>"
  Bus Selector/2 -> Send CAN Messages/2  "<IGN1>"
  Bus Selector/3 -> Send CAN Messages/3  "<dbgIGN2>"
  Bus Selector/4 -> Send CAN Messages/4  "<dbgCrank>"
  Bus Selector/5 -> Send CAN Messages/5  "<dbgShiftN>"
  Bus Selector/6 -> Send CAN Messages/6  "<dbgShiftR>"
  Bus Selector/7 -> Send CAN Messages/7  "<dbgShiftF>"
  Bus Selector/8 -> Send CAN Messages/8  "<sbgShiftErr>"
  Bus Selector/9 -> Send CAN Messages/9  "<BrakeSw>"
  Bus Selector/10 -> Send CAN Messages/10  "<DefrostSW>"
  Bus Selector/11 -> Send CAN Messages/11  "<WiperSw>"
  Bus Selector/12 -> Send CAN Messages/12  "<dbgAPPok>"
  Bus Selector/13 -> Send CAN Messages/13  "<csCANok>"
  Bus Selector/14 -> Send CAN Messages/14  "<CurrentFdbkOK>"
  Bus Selector/15 -> Send CAN Messages/15  "<CANchargerOK>"
  Bus Selector/16 -> Send CAN Messages/16  "<SOCok>"
  Bus Selector/17 -> Send CAN Messages/17  "<ErrorField>"
  Bus Selector/24 -> Send CAN Messages/24  "<VoltageFault>"
  Bus Selector/23 -> Send CAN Messages/23  "<CellVoltLow>"
  Bus Selector/22 -> Send CAN Messages/22  "<CellVoltHigh>"
  Bus Selector/21 -> Send CAN Messages/21  "<PackOverRegen>"
  Bus Selector/20 -> Send CAN Messages/20  "<PackOverCurrent>"
  Bus Selector/19 -> Send CAN Messages/19  "<PackVoltLow>"
  Bus Selector/18 -> Send CAN Messages/18  "<BatteryFault>"
  Bus Selector/25 -> Send CAN Messages/25  "<ReadyLight>"
  Bus Selector/26 -> Send CAN Messages/26  "<FaultMode>"
  Bus Selector/27 -> Send CAN Messages/27  "<DriveMode>"
  Bus Selector/28 -> Send CAN Messages/28  "<ChargeMode>"
  Bus Selector/29 -> Send CAN Messages/29  "<acPresent>"
  Bus Selector/30 -> Send CAN Messages/30  "<DBGinverterOT>"
  Bus Selector/31 -> Send CAN Messages/31  "<DBGmotorOT>"
  Bus Selector/32 -> Send CAN Messages/32  "<BatteryFault>"
  Bus Selector/33 -> Send CAN Messages/33  "<Charger Enabled>"
  Bus Selector/34 -> Send CAN Messages/34  "<ChargerOut>"
  Bus Selector/35 -> Send CAN Messages/35  "<PackBalanced>"
  Bus Selector/36 -> Send CAN Messages/36  "<PackCharging>"
  Bus Selector/37 -> Send CAN Messages/37  "<PackCooldown>"
  Bus Selector/38 -> Send CAN Messages/38  "<PackCharged>"
  Bus Selector/39 -> Send CAN Messages/39  "<CellDrained>"
  Bus Selector/40 -> Send CAN Messages/40  "<CellsCharged>"
  Bus Selector/41 -> Send CAN Messages/41  "<CellOver>"
  Bus Selector/42 -> Send CAN Messages/42  "<CellHigh>"
  Bus Selector/43 -> Send CAN Messages/43  "<ContactorFault>"
  Bus Selector/44 -> Send CAN Messages/44  "<SSCont>"
  Bus Selector/45 -> Send CAN Messages/45  "<MainCont>"
  Bus Selector/46 -> Send CAN Messages/46  "<HVaccRly>"

== system GTA_PCMFirmware/Function/3 Output and Debug/CAN/Debug/Message 0x701 ==
  In1 : Inport
  Bus Selector : BusSelector  OutputSignals=InputBus.CANin.Motor Controller.KinTempWarn.WarningFlags,InputBus.CANin.Motor Controller.KinVoltSpeed.ErrorField,InputBus.AnalogIn.ThrottlePedal.PedalPerc,InputBus.CANin.BMS.csInfo.csSOC
  Send CAN Messages : MotoHawk_lib/CAN Blocks/Send CAN Messages  bus=-2  nam='CAN_1'  msgl=CANMSG_Debug701  pace=5  labelwires=off
  wires:
  In1/1 -> Bus Selector/1
  Bus Selector/1 -> Send CAN Messages/1  "<WarningFlags>"
  Bus Selector/2 -> Send CAN Messages/2  "<ErrorField>"
  Bus Selector/3 -> Send CAN Messages/3  "<PedalPerc>"
  Bus Selector/4 -> Send CAN Messages/4  "<csSOC>"

== system GTA_PCMFirmware/Function/3 Output and Debug/CAN/Debug/Message 0x702 ==
  In1 : Inport
  Bus Selector : BusSelector  OutputSignals=InputBus.CANin.BMS.csCellInfo.PackVoltage,InputBus.CANin.BMS.csCellInfo.HighCellValue,InputBus.CANin.BMS.csCellInfo.LowCellValue,InputBus.CANin.Motor Controller.KinVoltSpeed.VoltageCap,InputBus.AnalogIn.SupplySense.12VSense
  Send CAN Messages : MotoHawk_lib/CAN Blocks/Send CAN Messages  bus=-2  nam='CAN_1'  msgl=CANMSG_Debug702  pace=5  labelwires=off
  wires:
  In1/1 -> Bus Selector/1
  Bus Selector/5 -> Send CAN Messages/5  "<12VSense>"
  Bus Selector/1 -> Send CAN Messages/1  "<PackVoltage>"
  Bus Selector/2 -> Send CAN Messages/2  "<HighCellValue>"
  Bus Selector/3 -> Send CAN Messages/3  "<LowCellValue>"
  Bus Selector/4 -> Send CAN Messages/4  "<VoltageCap>"

== system GTA_PCMFirmware/Function/3 Output and Debug/CAN/Debug/Message 0x703 ==
  In1 : Inport
  Bus Selector : BusSelector  OutputSignals=InputBus.CANin.BMS.csInfo.csCurrent,ControlBus.MotorControl.torqueRequest,InputBus.CANin.Motor Controller.KinCurrFB.iq_ref,InputBus.CANin.Motor Controller.KinCurrFB.iq_n
  Send CAN Messages : MotoHawk_lib/CAN Blocks/Send CAN Messages  bus=-2  nam='CAN_1'  msgl=CANMSG_Debug703  pace=5  labelwires=off
  wires:
  In1/1 -> Bus Selector/1
  Bus Selector/3 -> Send CAN Messages/3  "<iq_ref>"
  Bus Selector/4 -> Send CAN Messages/4  "<iq_n>"
  Bus Selector/1 -> Send CAN Messages/1  "<csCurrent>"
  Bus Selector/2 -> Send CAN Messages/2  "<torqueRequest>"

== system GTA_PCMFirmware/Function/3 Output and Debug/CAN/Debug/Message 0x704 ==
  In1 : Inport
  Bus Selector : BusSelector  OutputSignals=InputBus.CANin.BMS.csCellTemps.HighCellTemp,InputBus.CANin.BMS.csCellTemps.LowCellTemp,InputBus.CANin.BMS.csPackSize.PackSize
  Send CAN Messages : MotoHawk_lib/CAN Blocks/Send CAN Messages  bus=-2  nam='CAN_1'  msgl=CANMSG_Debug704  pace=5  labelwires=off
  wires:
  In1/1 -> Bus Selector/1
  Bus Selector/2 -> Send CAN Messages/2  "<LowCellTemp>"
  Bus Selector/1 -> Send CAN Messages/1  "<HighCellTemp>"
  Bus Selector/3 -> Send CAN Messages/3  "<PackSize>"

== system GTA_PCMFirmware/Function/3 Output and Debug/CAN/Instrument Cluster/MCU ==
  InputBus : Inport
  Abs : Abs
  Bus Selector : BusSelector  OutputSignals=CANin.Motor Controller.KinVoltSpeed.MotorSpeed
  Send CAN Messages : MotoHawk_lib/CAN Blocks/Send CAN Messages  bus=-2  nam='CAN_1'  msgl=CANMSG_ClusterMCU1  pace=5  labelwires=off
  motohawk_override_abs : MotoHawk_lib/Calibration & Probing Blocks/motohawk_override_abs  parent_name='MotorSpeed'  parent_val=0  show_more=off  name_source=Use Parameter  parent_read_level=1  parent_override_level=1  view_as=Number  enum_struct={'Disabled', 'Enabled'}  use_help_units=off  parent_help=''  parent_units=''  use_min_max=off  parent_min=-inf  parent_max=inf  use_precision=off  parent_precision=''  parent_gain=1  parent_offset=0  parent_exp=1  use_mototune_group=off  parent_group=motohawk_vardec_path(gcb)
  motohawk_probe : MotoHawk_lib/Calibration & Probing Blocks/motohawk_probe  nam='MotorSpeed'  show_more=off  name_source=Use Parameter  read_level=1  view_as=Number  enum_struct={'Disabled', 'Enabled'}  vector_style=Wide Row  use_help_units=off  help=''  units=''  use_header_enum=off  row_header_enum={}  col_header_enum={}  use_min_max=off  min_val=-inf  max_val=inf  use_precision=off  precision=''  gain=1  offset=0  exp=1  use_mototune_group=off  mototune_group=motohawk_vardec_path(gcb)
  wires:
  InputBus/1 -> Bus Selector/1
  Bus Selector/1 -> Abs/1  "<MotorSpeed>"
  Abs/1 -> motohawk_override_abs/1, motohawk_probe/1
  motohawk_override_abs/1 -> Send CAN Messages/1
